simulink model "ejemplo_arduino2"  (R2014b)
settings: Solver=ode3  StartTime=0.0  StopTime=inf  FixedStep=0.001  RelTol=1e-3
libraries: simulink x48, simulink_extras x36, dspswit3 x16, LibrarySimulinkSAS x2, vrlib x2, sldrtlib x1
(part 1 of 2)
settings Model: Creator=Usuario  LastModifiedBy=santd
settings OptimizationCC: UseDivisionForNetSlopeComputation=off  SimCompilerOptimization=off
settings DebuggingCC: FrameProcessingCompatibilityMsg=error
settings RTWCC: RTWCompilerOptimization=off
settings ConfigComp: CovMetricSettings=dw  CovHtmlReporting=on  CovSaveCumulativeToWorkspaceVar=on  CovSaveSingleToWorkspaceVar=on  CovModelRefEnable=Off  CovExternalEMLEnable=off  CovSFcnEnable=off
settings ConfigurationSet: Description=Simscape Multibody

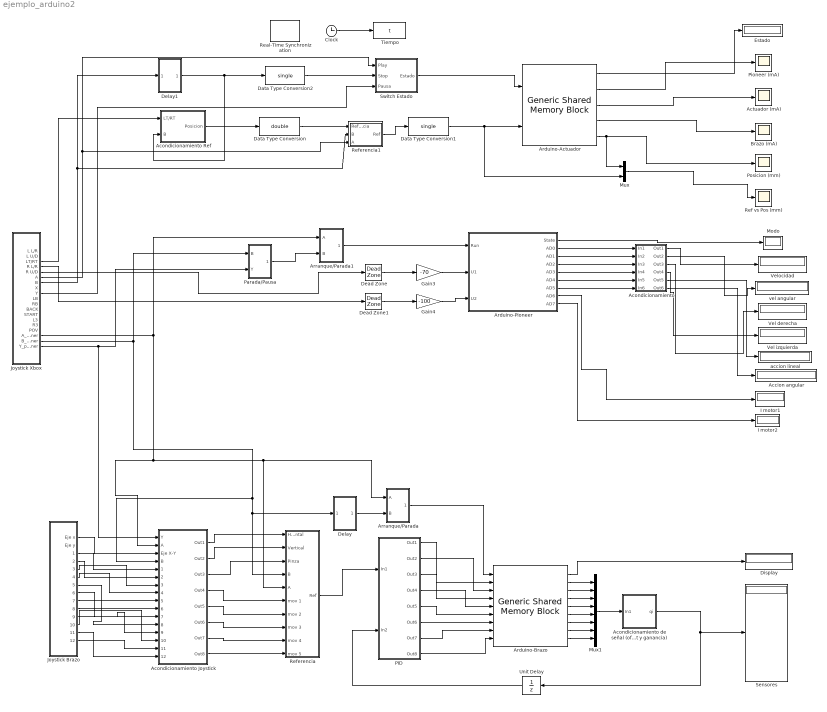
== system ejemplo_arduino2 ==
  Accion angular : Display
  "Acondicionamiento " : Subsystem
  Acondicionamiento Joystick : Subsystem
  Acondicionamiento Ref : Subsystem
  Acondicionamiento de señal (offset y ganancia) : Subsystem
  Actuador (mA) : Scope
      settings: YMin=0  YMax=2000
  Arduino-Actuador : LibrarySimulinkSAS/Generic Shared Memory Block  nombre='memoriaEjemplo'  dispositivo=10  vecE=[3 2 1]  vecS=[4 5 6 156]  tipoE=['f' 'I' 'c']  tipoS=['C' 'i' 'd' 'd']
  Arduino-Brazo : LibrarySimulinkSAS/Generic Shared Memory Block  nombre='memoriaEjemplo'  dispositivo=10  vecE=[3 2 1]  vecS=[4 5 6 156]  tipoE=['f' 'I' 'c']  tipoS=['C' 'i' 'd' 'd']
  Arduino-Pioneer : Subsystem  mask{dev=3}
      mask prompts: dev "Device Number"
      mask Help:
      | HELP DEVICE
      | 
      | - App for using the kit arduino UNO plus Adafruit motor shield 1.2 based on two L293D chips forming 4 H-Bridges. L293D chipset provides 0.6A per bridge (1.2A peak) with thermal shutdown protection, internal kickback protection diodes. Can run motors on 4.5VDC to 25VDC. The shield is compatible with Arduino Mega 1280 & 2560, Diecimila, Duemilanove, and UNO
      | 
      | HELP DRIVERS
      | 
      | Upload the firmware 'Arduino_motor_firmware' in your Arduino UNO kit available from folder '\SAS TOOLS\Software arduino_motor V1.1.0'
      | -------------------------------------------------------------------------------------------------------------------------------------------------------
      | HELP APP
      | 
      | Before running the Simulink model initiate communication with the device through the application 'Arduino_motor.exe' available from folder '\SAS TOOLS\Software arduino_motor V1.1.0'. After executing the program the app icon is available in the taskbar.
      | The app "arduino_motor.exe" is handled from right-click on the icon and selecting the corresponding option:
      | "Play" -> Start the commnunication between the device and the app
      | "Stop" -> Stop the communication
      | "Monitor"->view the state of sensors and communication
      | 
      | -------------------------------------------------------------------------------------------------------------------------------------------------------
      | 
      | HELP BLOCK
      | 
      | Input Ports
      | 
      | Port 'Run': 1 for running and 0 for stopping
      | 
      | Port 'U1': value between [-255;255] which drives the tension applied to the motor 1 of the shield motor Adafruit 1.0
      | Port 'U2': value between [-255;255] which drives the tension applied to the motor 2 of the shield motor Adafruit 1.0
      | Port 'U3': value between [-255;255] which drives the tension applied to the motor 3 of the shield motor Adafruit 1.0
      | Port 'U4': value between [-255;255] which drives the tension applied to the motor 4 of the shield motor Adafruit 1.0
      | 
      | The range [-255;255] is related with the tension range [-V;V], where V is the tension source applied to the motor shield
      | 
      | Output Ports
      | 
      | Port 'State': information about the system. Run=1; Stop=0
      | 
      | Port 'AD0': value between [0;1023] measured in the pin AD0 of the Arduino UNO board
      | Port 'AD1': value between [0;1023] measured in the pin AD1 of the Arduino UNO board
      | Port 'AD2': value between [0;1023] measured in the pin AD2 of the Arduino UNO board
      | Port 'AD3': value between [0;1023] measured in the pin AD3 of the Arduino UNO board
      | 
      | The range [0;1023] is related with the tension range [0;5V] readed on the pins of the Arduino kit A/D conversor
      | -------------------------------------------------------------------------------------------------------------------------------------------------------
      | 
      | HELP SHARE MEMORY (information only for external applications different to "Arduino_motor.exe")
      | 
      | Shared Memory Names:
      | 
      | 'ARDUINO_entrada_'#dev
      | 'ARDUINO_salida_'#dev
      | NOTE: replace #dev with the device number
      mask DialogControl DescGroupVar Prompt: Arduino motor shield
      mask DialogControl DescTextVar Prompt: This block is used to receive and send data via USB port between a UNO Arduino board and the App "Arduino_motor.exe" available on folder '\SAS TOOLS\Software Arduino_motor V1.1.0'. You must upload the firmware "Arduino_motor_firmware" into your Arduino board. More information in Help button.
      mask Display:
      | image('motor_shield.png')
      | color('red')
      | port_label('input',1,'run')
      | port_label('input',2,'U1')
      | port_label('input',3,'U2')
      | port_label('input',4,'U3')
      | port_label('input',5,'U4')
      | color('blue')
      | port_label('output',1,'state')
      | port_label('output',2,'AD0')
      | port_label('output',3,'AD1')
      | port_label('output',4,'AD2')
      | port_label('output',5,'AD3')
  Arranque/Parada : Subsystem
  Arranque/Parada1 : Subsystem
  Brazo (mA) : Scope
      settings: YMin=0  YMax=2000
  Clock : Clock
  Data Type Conversion : DataTypeConversion  OutDataTypeStr=double
  Data Type Conversion1 : DataTypeConversion  OutDataTypeStr=single
  Data Type Conversion2 : DataTypeConversion  OutDataTypeStr=single
  Dead Zone : DeadZone  LowerValue=-0.2  UpperValue=0.2  SaturateOnIntegerOverflow=on
  Dead Zone1 : DeadZone  LowerValue=-0.2  UpperValue=0.2  SaturateOnIntegerOverflow=on
  Delay : Subsystem
  Delay1 : Subsystem
  Display : Display
  Estado : Display
  Gain3 : Gain  Gain=-70  OutDataTypeStr=single
  Gain4 : Gain  Gain=-100  OutDataTypeStr=single
  I motor1 : Display
  I motor2 : Display
  Joystick Brazo : Subsystem
  Joystick Xbox : Subsystem
  Modo : Display
  Mux : Mux  Inputs=2
  Mux1 : Mux  Inputs=8
  PID : Subsystem
  Parada/Pausa : Subsystem
  Pioneer (mA) : Scope
      settings: YMin=0  YMax=2500
  Posicion (mm) : Scope
      settings: YMin=-10  YMax=220
  Real-Time Synchronization : sldrtlib/Real-Time Synchronization
  Ref vs Pos (mm) : Scope
      settings: YMin=0  YMax=200
  Referencia : Subsystem
  Referencia1 : Subsystem
  Sensores : Display
  Switch Estado : Subsystem
  Tiempo : ToWorkspace  VariableName=t  SampleTime=-1
  Unit Delay : UnitDelay  SampleTime=-1
  Vel derecha : Display
  Vel izquierda : Display
  Velocidad : Display
  accion lineal : Display
  vel angular : Display
  wires:
  Clock/1 -> Tiempo/1
  Arduino-Actuador/1 -> Estado/1
  Arduino-Actuador/2 -> Pioneer (mA)/1
  Arduino-Actuador/3 -> Actuador (mA)/1
  Arduino-Actuador/4 -> Brazo (mA)/1
  Joystick Xbox/6(A) -> Referencia1/3(A), Switch Estado/1(Play)
  Joystick Xbox/9(Y) -> Switch Estado/3(Pausa)
  Switch Estado/1(Estado) -> Arduino-Actuador/1
  Arduino-Brazo/1 -> Display/1
  Arduino-Brazo/2 -> Mux1/1
  Arduino-Brazo/9 -> Mux1/8
  Arduino-Brazo/7 -> Mux1/6
  Arduino-Brazo/8 -> Mux1/7
  Arduino-Brazo/6 -> Mux1/5
  Arduino-Brazo/3 -> Mux1/2
  Arduino-Brazo/4 -> Mux1/3
  Arduino-Brazo/5 -> Mux1/4
  Mux1/1 -> Acondicionamiento de señal (offset y ganancia)/1(In1)
  Acondicionamiento de señal (offset y ganancia)/1(qi) -> Unit Delay/1, Sensores/1
  Referencia/1(Ref) -> PID/1(In1)
  Joystick Xbox/17(A_Pionner) -> Arranque/Parada1/1(A), Referencia/5(A), Arranque/Parada/1(A), Acondicionamiento Joystick/2(A)
  Joystick Xbox/18(B_Pionner) -> Parada/Pausa/1(B), Referencia/4(B), Delay/1(In1), Acondicionamiento Joystick/4(B)
  Joystick Xbox/19(Y_pionner) -> Acondicionamiento Joystick/1(Y), Parada/Pausa/2(Y)
  Gain4/1 -> Arduino-Pioneer/3(U2)
  Arduino-Pioneer/1(State) -> Modo/1
  Arranque/Parada1/1(Modo) -> Arduino-Pioneer/1(Run)
  Gain3/1 -> Arduino-Pioneer/2(U1)
  Arduino-Pioneer/8(AD6) -> I motor1/1
  Arduino-Pioneer/9(AD7) -> I motor2/1
  Unit Delay/1 -> PID/2(In2)
  PID/1(Out1) -> Arduino-Brazo/2
  PID/2(Out2) -> Arduino-Brazo/3
  PID/3(Out3) -> Arduino-Brazo/4
  PID/4(Out4) -> Arduino-Brazo/5
  PID/5(Out5) -> Arduino-Brazo/6
  PID/6(Out6) -> Arduino-Brazo/7
  PID/7(Out7) -> Arduino-Brazo/8
  PID/8(Out8) -> Arduino-Brazo/9
  Parada/Pausa/1(Out1) -> Arranque/Parada1/2(B)
  Arduino-Pioneer/2(AD0) -> "Acondicionamiento "/1(In1)
  Arduino-Pioneer/3(AD1) -> "Acondicionamiento "/2(In2)
  Arduino-Pioneer/4(AD2) -> "Acondicionamiento "/3(In3)
  Arduino-Pioneer/5(AD3) -> "Acondicionamiento "/4(In4)
  Arduino-Pioneer/6(AD4) -> "Acondicionamiento "/5(In5)
  Arduino-Pioneer/7(AD5) -> "Acondicionamiento "/6(In6)
  "Acondicionamiento "/1(Out1) -> Velocidad/1
  "Acondicionamiento "/2(Out2) -> vel angular/1
  "Acondicionamiento "/3(Out3) -> Vel derecha/1
  "Acondicionamiento "/4(Out4) -> Vel izquierda/1
  "Acondicionamiento "/5(Out5) -> accion lineal/1
  "Acondicionamiento "/6(Out6) -> Accion angular/1
  Arranque/Parada/1(Modo) -> Arduino-Brazo/1
  Delay/1(Out1) -> Arranque/Parada/2(B)
  Joystick Brazo/1(Eje x) -> Acondicionamiento Joystick/3(Eje X-Y)
  Joystick Brazo/3(1) -> Acondicionamiento Joystick/5(1)
  Joystick Brazo/4(2) -> Acondicionamiento Joystick/6(2)
  Joystick Brazo/5(3) -> Acondicionamiento Joystick/7(3)
  Joystick Brazo/6(4) -> Acondicionamiento Joystick/8(4)
  Joystick Brazo/11(9) -> Acondicionamiento Joystick/13(9)
  Joystick Brazo/12(10) -> Acondicionamiento Joystick/14(10)
  Acondicionamiento Joystick/1(Out1) -> Referencia/1(Horizontal)
  Acondicionamiento Joystick/2(Out2) -> Referencia/2(Vertical)
  Acondicionamiento Joystick/3(Out3) -> Referencia/3(Pinza)
  Acondicionamiento Joystick/4(Out4) -> Referencia/6(mov 1)
  Acondicionamiento Joystick/5(Out5) -> Referencia/7(mov 2)
  Acondicionamiento Joystick/6(Out6) -> Referencia/8(mov 3)
  Acondicionamiento Joystick/7(Out7) -> Referencia/9(mov 4)
  Acondicionamiento Joystick/8(Out8) -> Referencia/10(mov 5)
  Joystick Brazo/9(7) -> Acondicionamiento Joystick/9(5)
  Joystick Brazo/10(8) -> Acondicionamiento Joystick/10(6)
  Joystick Brazo/7(5) -> Acondicionamiento Joystick/12(8)
  Joystick Brazo/8(6) -> Acondicionamiento Joystick/11(7)
  Joystick Brazo/13(11) -> Acondicionamiento Joystick/16(12)
  Joystick Brazo/14(12) -> Acondicionamiento Joystick/15(11)
  Dead Zone1/1 -> Gain4/1
  Dead Zone/1 -> Gain3/1
  Joystick Xbox/4(R L/R) -> Dead Zone1/1
  Joystick Xbox/5(R U/D) -> Dead Zone/1
  Arduino-Actuador/5 -> Posicion (mm)/1, Mux/1
  Joystick Xbox/3(LT/RT) -> Acondicionamiento Ref/1(LT/RT)
  Referencia1/1(Ref) -> Data Type Conversion1/1
  Mux/1 -> Ref vs Pos (mm)/1
  Acondicionamiento Ref/1(Posicion) -> Data Type Conversion/1
  Data Type Conversion/1 -> Referencia1/1(Referencia)
  Data Type Conversion1/1 -> Mux/2, Arduino-Actuador/2
  Joystick Xbox/7(B) -> Delay1/1(In1), Referencia1/2(B)
  Data Type Conversion2/1 -> Switch Estado/2(Stop)
  Delay1/1(Out1) -> Acondicionamiento Ref/2(B), Data Type Conversion2/1

== system ejemplo_arduino2/Acondicionamiento  ==
  In1 : Inport
  In2 : Inport  Port=2
  In3 : Inport  Port=3
  In4 : Inport  Port=4
  In5 : Inport  Port=5
  In6 : Inport  Port=6
  Subsystem : Subsystem
  Subsystem1 : Subsystem
  Subsystem2 : Subsystem
  Subsystem3 : Subsystem
  Subsystem4 : Subsystem
  Subsystem5 : Subsystem
  Out1 : Outport
  Out2 : Outport  Port=2
  Out3 : Outport  Port=3
  Out4 : Outport  Port=4
  Out5 : Outport  Port=5
  Out6 : Outport  Port=6
  wires:
  In4/1 -> Subsystem2/1(In1)
  In3/1 -> Subsystem1/1(In1)
  In2/1 -> Subsystem3/1(In1)
  Subsystem5/1(Out1) -> Out6/1
  In6/1 -> Subsystem5/1(In1)
  Subsystem4/1(Out1) -> Out5/1
  In5/1 -> Subsystem4/1(In1)
  Subsystem2/1(Out1) -> Out4/1
  Subsystem3/1(Out1) -> Out2/1
  Subsystem1/1(Out1) -> Out3/1
  Subsystem/1(Out1) -> Out1/1
  In1/1 -> Subsystem/1(In1)

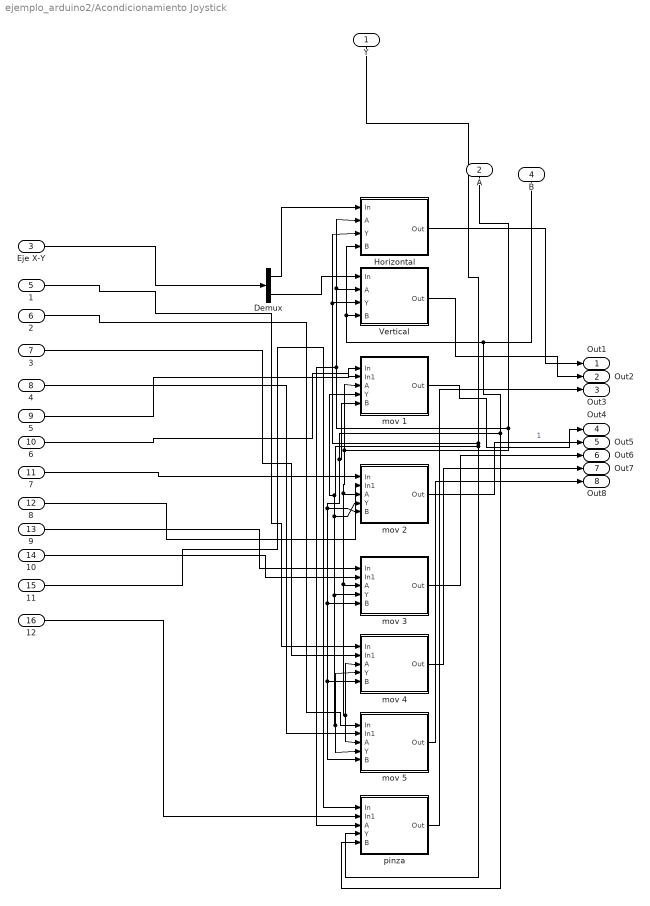
== system ejemplo_arduino2/Acondicionamiento Joystick ==
  Y : Inport
  A : Inport  Port=2
  Eje X-Y : Inport  Port=3
  B : Inport  Port=4
  1 : Inport  Port=5
  2 : Inport  Port=6
  3 : Inport  Port=7
  4 : Inport  Port=8
  5 : Inport  Port=9
  6 : Inport  Port=10
  7 : Inport  Port=11
  8 : Inport  Port=12
  9 : Inport  Port=13
  10 : Inport  Port=14
  11 : Inport  Port=15
  12 : Inport  Port=16
  Demux : Demux  Outputs=2
  Horizontal : Subsystem
  Vertical : Subsystem
  mov 1 : Subsystem
  mov 2 : Subsystem
  mov 3 : Subsystem
  mov 4 : Subsystem
  mov 5 : Subsystem
  pinza : Subsystem
  Out1 : Outport
  Out2 : Outport  Port=2
  Out3 : Outport  Port=3
  Out4 : Outport  Port=4
  Out5 : Outport  Port=5
  Out6 : Outport  Port=6
  Out7 : Outport  Port=7
  Out8 : Outport  Port=8
  wires:
  pinza/1(Out) -> Out3/1
  Eje X-Y/1 -> Demux/1
  11/1 -> pinza/1(In)
  12/1 -> pinza/2(In1)
  mov 1/1(Out) -> Out4/1
  mov 2/1(Out) -> Out5/1  "1"
  mov 3/1(Out) -> Out6/1
  mov 4/1(Out) -> Out7/1
  5/1 -> mov 1/1(In)
  6/1 -> mov 1/2(In1)
  7/1 -> mov 2/1(In)
  8/1 -> mov 2/2(In1)
  9/1 -> mov 3/1(In)
  10/1 -> mov 3/2(In1)
  mov 5/1(Out) -> Out8/1
  Horizontal/1(Out) -> Out1/1
  Vertical/1(Out) -> Out2/1
  Demux/1 -> Horizontal/1(In)
  Demux/2 -> Vertical/1(In)
  1/1 -> mov 4/1(In)
  3/1 -> mov 4/2(In1)
  2/1 -> mov 5/1(In)
  4/1 -> mov 5/2(In1)
  Y/1 -> pinza/4(Y), mov 5/4(Y), mov 4/4(Y), mov 3/4(Y), mov 2/4(Y), mov 1/4(Y), Horizontal/3(Y), Vertical/3(Y)
  A/1 -> Horizontal/2(A), Vertical/2(A), pinza/3(A), mov 5/3(A), mov 4/3(A), mov 3/3(A), mov 2/3(A), mov 1/3(A)
  B/1 -> Horizontal/4(B), Vertical/4(B), mov 5/5(B), mov 4/5(B), mov 3/5(B), mov 2/5(B), mov 1/5(B), pinza/5(B)

== system ejemplo_arduino2/Acondicionamiento Ref ==
  LT/RT : Inport
  B : Inport  Port=2
  Constant : Constant  Value=0
  Data Type Conversion : DataTypeConversion
  Data Type Conversion1 : DataTypeConversion  OutDataTypeStr=single
  Gain : Gain  Gain=-26  OutDataTypeStr=single
  Integrator Limited : Integrator  ExternalReset=level  InitialConditionSource=external  LimitOutput=on  UpperSaturationLimit=200  LowerSaturationLimit=0
  Posicion : Outport
  wires:
  LT/RT/1 -> Gain/1
  Gain/1 -> Data Type Conversion/1
  Data Type Conversion/1 -> Integrator Limited/1
  Integrator Limited/1 -> Data Type Conversion1/1
  Data Type Conversion1/1 -> Posicion/1
  B/1 -> Integrator Limited/2
  Constant/1 -> Integrator Limited/3

== system ejemplo_arduino2/Acondicionamiento de señal (offset y ganancia) ==
  In1 : Inport
  Ganancia : Gain  Gain=diag([0.2022 0.2057 0.2093 0.2047 0.2179 0.2024 0.1931 0.3141])  Multiplication=Matrix(K*u) (u vector)
  Offset : Constant  Value=[-132 -113 -162 -88 -125 -124 -90 -386]
  Sum : Sum  Inputs=|++
  qi : Outport
  wires:
  In1/1 -> Sum/1
  Sum/1 -> Ganancia/1
  Offset/1 -> Sum/2
  Ganancia/1 -> qi/1

== system ejemplo_arduino2/Arduino-Pioneer ==
  Run : Inport
  U1 : Inport  Port=2
  U2 : Inport  Port=3
  Generic Shared Memory Block : S-Function  FunctionName=matlabGenericSHM  Parameters=nombre,dispositivo,vecE,vecS,tipoE,tipoS  EnableBusSupport=off  mask(Generic Share Memory block V2.0){nombre='ARDUINO', dispositivo=3, vecE=[1 1 1], vecS=[1 1 1 1 1 1 1 1 1], tipoE=['f' 'f' 'f'], tipoS=['f' 'f' 'f' 'f' 'f' 'f' 'f' 'f' 'f' ]}
      mask prompts: nombre "Share Memory base name"; dispositivo "Device Number"; vecE "Sizes input vector"; vecS "Sizes output vector"; tipoE "Data Types Inputs"; tipoS "Data Types Outputs"
      mask help:
      | This block allows Simulink communication with external processes through shared memory. It works on Unix and Windows.
      | More information in Help.
      mask Help:
      | Share Memory base name (nombre): It's the base string of share memory ej 'robot'
      | Device Number (dispositivo): integer that identifies the device between multiple in use
      | Two shared memorys are created with names:
      | "%name_entrada_%dispositivo" for the device input (writing)
      | "%name_salida_%dispositivo" for the device output (reading)
      | Sizes input vector (vecE)  : array that specify the number of inputs (array dimension) and the inputs size (array values)
      | Sizes output vector  (vecS): array that specify the number of outputs (array dimension) and the outputs size (array values)
      | Data types input(tipoE): char array that specify each input types
      | Data types output (tipoS): char array that specify each output types
      | Allowed types are:
      | ('f'=float, 'd'=double, 'i'=int32, 'c'=char, 'C'= unsigned char, 'I'=unsigned int)
      | Example.
      | Suppose the following parameters:
      | nombre='exampleMemory'
      | dispositivo=10
      | vecE=[3 2 1]
      | vecS=[6 5 7 8]
      | tipoE=['f' 'I' 'c']
      | tipoS=['C' 'i' 'd' 'd']
      | 
      | Two Share Memories are created with names:
      | "exampleMemory_entrada_10" (block input)
      | "exampleMemory_salida_10"  (block output)
      | 3 inputs are created:
      |  1° Dimension 3, type "unsigned char"
      |  2° Dimension 2, type "int"
      |  3° Dimension 1, type "char"
      | 4 outputs are created:
      |  1° Dimension 6, type "float"
      |  2° Dimension 5, type "unsigned int"
      |  3° Dimension 7, type "double"
      |  3° Dimension 8, type "double"
      mask Display: image('shmem.jpg')
  State : Outport
  AD0 : Outport  Port=2
  AD1 : Outport  Port=3
  AD2 : Outport  Port=4
  AD3 : Outport  Port=5
  AD4 : Outport  Port=6
  AD5 : Outport  Port=7
  AD6 : Outport  Port=8
  AD7 : Outport  Port=9
  wires:
  Generic Shared Memory Block/5 -> AD3/1
  Generic Shared Memory Block/4 -> AD2/1
  Generic Shared Memory Block/3 -> AD1/1
  Generic Shared Memory Block/2 -> AD0/1
  Generic Shared Memory Block/1 -> State/1
  U2/1 -> Generic Shared Memory Block/3
  U1/1 -> Generic Shared Memory Block/2
  Run/1 -> Generic Shared Memory Block/1
  Generic Shared Memory Block/9 -> AD7/1
  Generic Shared Memory Block/8 -> AD6/1
  Generic Shared Memory Block/7 -> AD5/1
  Generic Shared Memory Block/6 -> AD4/1

== system ejemplo_arduino2/Arranque//Parada ==
  A : Inport
  B : Inport  Port=2
  Data Type Conversion2 : DataTypeConversion  OutDataTypeStr=single
  Detect Rise Positive : simulink/Logic and Bit Operations/Detect Rise Positive  vinit=0  InputProcessing=Inherited  OutDataTypeStr=boolean
  Detect Rise Positive1 : simulink/Logic and Bit Operations/Detect Rise Positive  vinit=0  InputProcessing=Inherited  OutDataTypeStr=boolean
  Entrada : Display
  S-R Flip-Flop : simulink_extras/Flip Flops/S-R Flip-Flop  initial_condition=0
  Modo : Outport
  wires:
  B/1 -> Detect Rise Positive1/1
  S-R Flip-Flop/1 -> Entrada/1, Data Type Conversion2/1
  Detect Rise Positive/1 -> S-R Flip-Flop/1
  Data Type Conversion2/1 -> Modo/1
  Detect Rise Positive1/1 -> S-R Flip-Flop/2
  A/1 -> Detect Rise Positive/1

== system ejemplo_arduino2/Arranque//Parada1 ==
  A : Inport
  B : Inport  Port=2
  Data Type Conversion2 : DataTypeConversion  OutDataTypeStr=single
  Detect Rise Positive : simulink/Logic and Bit Operations/Detect Rise Positive  vinit=0  InputProcessing=Inherited  OutDataTypeStr=boolean
  Detect Rise Positive1 : simulink/Logic and Bit Operations/Detect Rise Positive  vinit=0  InputProcessing=Inherited  OutDataTypeStr=boolean
  Entrada : Display
  S-R Flip-Flop : simulink_extras/Flip Flops/S-R Flip-Flop  initial_condition=0
  Modo : Outport
  wires:
  B/1 -> Detect Rise Positive1/1
  S-R Flip-Flop/1 -> Entrada/1, Data Type Conversion2/1
  Detect Rise Positive/1 -> S-R Flip-Flop/1
  Data Type Conversion2/1 -> Modo/1
  Detect Rise Positive1/1 -> S-R Flip-Flop/2
  A/1 -> Detect Rise Positive/1

== system ejemplo_arduino2/Delay ==
  In1 : Inport
  Data Type Conversion : DataTypeConversion
  Data Type Conversion1 : DataTypeConversion
  Transport Delay : TransportDelay  DelayTime=2  InitialOutput=1
  Out1 : Outport
  wires:
  In1/1 -> Data Type Conversion/1
  Data Type Conversion/1 -> Transport Delay/1
  Transport Delay/1 -> Data Type Conversion1/1
  Data Type Conversion1/1 -> Out1/1

== system ejemplo_arduino2/Delay1 ==
  In1 : Inport
  Data Type Conversion : DataTypeConversion
  Data Type Conversion1 : DataTypeConversion
  Transport Delay : TransportDelay  DelayTime=4  InitialOutput=1
  Out1 : Outport
  wires:
  In1/1 -> Data Type Conversion/1
  Data Type Conversion/1 -> Transport Delay/1
  Transport Delay/1 -> Data Type Conversion1/1
  Data Type Conversion1/1 -> Out1/1

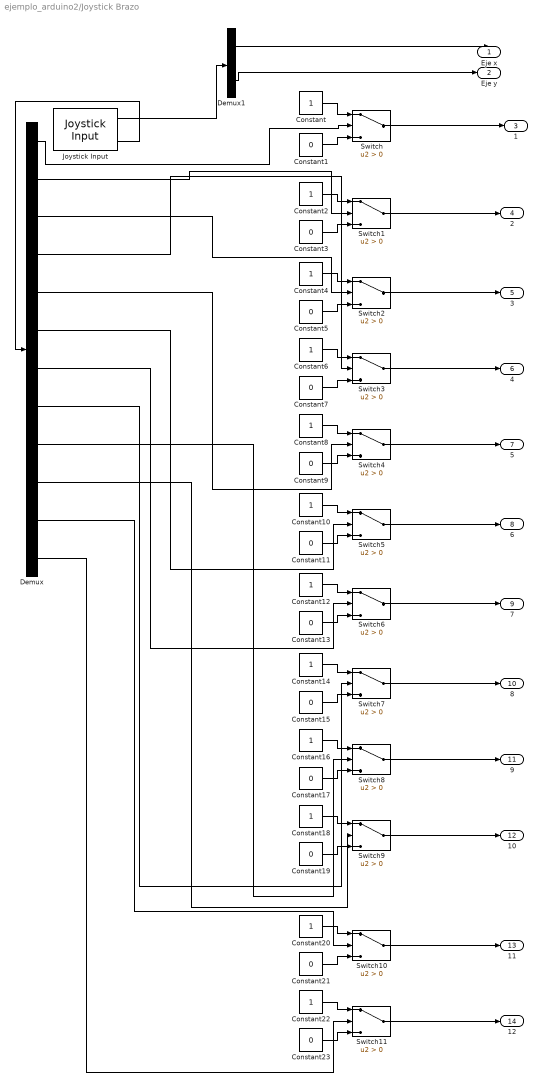
== system ejemplo_arduino2/Joystick Brazo ==
  Constant{,2,4,6,8,10,12,14,16,18,20,22} (12 alike) : Constant
  Constant{1,3,5,7,9,11,13,15,17,19,21,23} (12 alike) : Constant  Value=0
  Demux : Demux  Outputs=12
  Demux1 : Demux  Outputs=2
  Joystick Input : vrlib/Joystick Input  joyid=1  adjustports=off  forcefeed=off
  Switch{,1..11} (12 alike) : Switch  Criteria=u2 > Threshold  OutDataTypeStr=single  InputSameDT=on
  Eje x : Outport
  Eje y : Outport  Port=2
  1 : Outport  Port=3
  2 : Outport  Port=4
  3 : Outport  Port=5
  4 : Outport  Port=6
  5 : Outport  Port=7
  6 : Outport  Port=8
  7 : Outport  Port=9
  8 : Outport  Port=10
  9 : Outport  Port=11
  10 : Outport  Port=12
  11 : Outport  Port=13
  12 : Outport  Port=14
  wires:
  Joystick Input/2 -> Demux/1
  Demux/4 -> Switch3/2
  Demux/5 -> Switch4/2
  Constant16/1 -> Switch8/1
  Constant18/1 -> Switch9/1
  Demux/2 -> Switch1/2
  Switch9/1 -> 10/1
  Constant19/1 -> Switch9/3
  Switch8/1 -> 9/1
  Constant17/1 -> Switch8/3
  Demux/1 -> Switch/2
  Constant6/1 -> Switch3/1
  Constant3/1 -> Switch1/3
  Demux1/1 -> Eje x/1
  Demux/10 -> Switch9/2
  Demux/9 -> Switch8/2
  Switch2/1 -> 3/1
  Constant14/1 -> Switch7/1
  Switch7/1 -> 8/1
  Constant2/1 -> Switch1/1
  Constant5/1 -> Switch2/3
  Demux/8 -> Switch7/2
  Demux/7 -> Switch6/2
  Switch1/1 -> 2/1
  Constant4/1 -> Switch2/1
  Constant15/1 -> Switch7/3
  Constant7/1 -> Switch3/3
  Switch3/1 -> 4/1
  Demux/3 -> Switch2/2
  Constant10/1 -> Switch5/1
  Switch6/1 -> 7/1
  Switch5/1 -> 6/1
  Constant12/1 -> Switch6/1
  Constant13/1 -> Switch6/3
  Demux/6 -> Switch5/2
  Constant11/1 -> Switch5/3
  Switch/1 -> 1/1
  Constant8/1 -> Switch4/1
  Demux1/2 -> Eje y/1
  Constant9/1 -> Switch4/3
  Switch4/1 -> 5/1
  Constant1/1 -> Switch/3
  Constant/1 -> Switch/1
  Joystick Input/1 -> Demux1/1
  Constant20/1 -> Switch10/1
  Constant22/1 -> Switch11/1
  Switch11/1 -> 12/1
  Constant23/1 -> Switch11/3
  Switch10/1 -> 11/1
  Constant21/1 -> Switch10/3
  Demux/11 -> Switch10/2
  Demux/12 -> Switch11/2

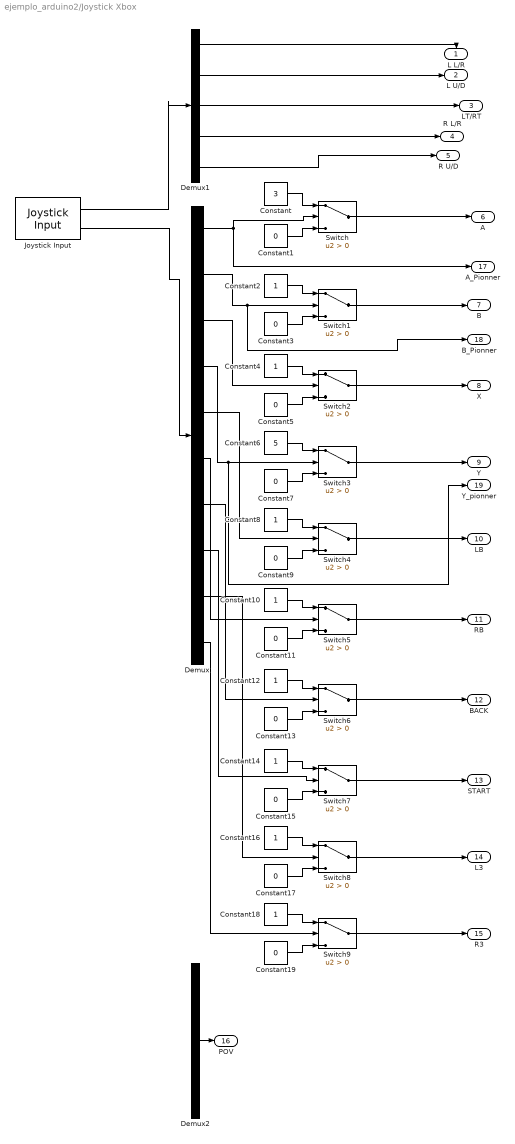
== system ejemplo_arduino2/Joystick Xbox ==
  Constant : Constant  Value=3
  Constant{1,3,5,7,9,11,13,15,17,19} (10 alike) : Constant  Value=0
  Constant{2,4,8,10,12,14,16,18} (8 alike) : Constant
  Constant6 : Constant  Value=5
  Demux : Demux  Outputs=10
  Demux1 : Demux  Outputs=5
  Demux2 : Demux  Outputs=1
  Joystick Input : vrlib/Joystick Input  joyid=1  adjustports=off  forcefeed=off
  Switch{,1..9} (10 alike) : Switch  Criteria=u2 > Threshold  OutDataTypeStr=single  InputSameDT=on
  L L/R : Outport
  L U/D : Outport  Port=2
  LT/RT : Outport  Port=3
  R L/R : Outport  Port=4
  R U/D : Outport  Port=5
  A : Outport  Port=6
  B : Outport  Port=7
  X : Outport  Port=8
  Y : Outport  Port=9
  LB : Outport  Port=10
  RB : Outport  Port=11
  BACK : Outport  Port=12
  START : Outport  Port=13
  L3 : Outport  Port=14
  R3 : Outport  Port=15
  POV : Outport  Port=16
  A_Pionner : Outport  Port=17
  B_Pionner : Outport  Port=18
  Y_pionner : Outport  Port=19
  wires:
  Joystick Input/2 -> Demux/1
  Demux2/1 -> POV/1
  ? -> Demux2/1
  Demux/4 -> Y_pionner/1, Switch3/2
  Demux/5 -> Switch4/2
  Constant16/1 -> Switch8/1
  Demux1/4 -> R L/R/1
  Constant18/1 -> Switch9/1
  Demux/2 -> B_Pionner/1, Switch1/2
  Switch9/1 -> R3/1
  Constant19/1 -> Switch9/3
  Switch8/1 -> L3/1
  Constant17/1 -> Switch8/3
  Demux/1 -> A_Pionner/1, Switch/2
  Demux1/5 -> R U/D/1
  Constant6/1 -> Switch3/1
  Constant3/1 -> Switch1/3
  Demux1/1 -> L L/R/1
  Demux/10 -> Switch9/2
  Demux/9 -> Switch8/2
  Switch2/1 -> X/1
  Constant14/1 -> Switch7/1
  Switch7/1 -> START/1
  Constant2/1 -> Switch1/1
  Constant5/1 -> Switch2/3
  Demux/8 -> Switch7/2
  Demux/7 -> Switch6/2
  Switch1/1 -> B/1
  Constant4/1 -> Switch2/1
  Constant15/1 -> Switch7/3
  Constant7/1 -> Switch3/3
  Switch3/1 -> Y/1
  Demux/3 -> Switch2/2
  Constant10/1 -> Switch5/1
  Switch6/1 -> BACK/1
  Switch5/1 -> RB/1
  Constant12/1 -> Switch6/1
  Constant13/1 -> Switch6/3
  Demux/6 -> Switch5/2
  Constant11/1 -> Switch5/3
  Switch/1 -> A/1
  Constant8/1 -> Switch4/1
  Demux1/2 -> L U/D/1
  Constant9/1 -> Switch4/3
  Switch4/1 -> LB/1
  Constant1/1 -> Switch/3
  Constant/1 -> Switch/1
  Joystick Input/1 -> Demux1/1
  Demux1/3 -> LT/RT/1

== system ejemplo_arduino2/PID ==
  In1 : Inport
  In2 : Inport  Port=2
  Demux : Demux  Outputs=8
  PID Controller{1..8} (8 alike) : simulink/Continuous/PID Controller  Controller=PID  TimeDomain=Continuous-time  SampleTime=-1  IntegratorMethod=Forward Euler  FilterMethod=Forward Euler  Form=Parallel  P=1  I=1  D=0  N=100  InitialConditionSource=internal  InitialConditionForIntegrator=0  InitialConditionForFilter=0  ExternalReset=none  LimitOutput=off  UpperSaturationLimit=inf  LowerSaturationLimit=-inf  LinearizeAsGain=on  AntiWindupMode=none  Kb=1  TrackingMode=off  Kt=1  PParamMin=[]  PParamMax=[]  IParamMin=[]  IParamMax=[]  DParamMin=[]  DParamMax=[]  NParamMin=[]  NParamMax=[]  KbParamMin=[]  KbParamMax=[]  KtParamMin=[]  KtParamMax=[]  POutMin=[]  POutMax=[]  IOutMin=[]  IOutMax=[]  DOutMin=[]  DOutMax=[]  NOutMin=[]  NOutMax=[]  KbOutMin=[]  KbOutMax=[]  KtOutMin=[]  KtOutMax=[]  IntegratorOutMin=[]  IntegratorOutMax=[]  FilterOutMin=[]  FilterOutMax=[]  SumOutMin=[]  SumOutMax=[]  SumI1OutMin=[]  SumI1OutMax=[]  SumI2OutMin=[]  SumI2OutMax=[]  SumI3OutMin=[]  SumI3OutMax=[]  SumDOutMin=[]  SumDOutMax=[]  SaturationOutMin=[]  SaturationOutMax=[]  IntegratorContinuousStateAttributes=''  IntegratorStateMustResolveToSignalObject=off  IntegratorRTWStateStorageClass=Auto  FilterContinuousStateAttributes=''  FilterStateMustResolveToSignalObject=off  FilterRTWStateStorageClass=Auto  DifferentiatorICPrevScaledInput=0  DifferentiatorOutMin=[]  DifferentiatorOutMax=[]  UseFilter=on
  Subtract1 : Sum  Inputs=+-
  Out1 : Outport
  Out2 : Outport  Port=2
  Out3 : Outport  Port=3
  Out4 : Outport  Port=4
  Out5 : Outport  Port=5
  Out6 : Outport  Port=6
  Out7 : Outport  Port=7
  Out8 : Outport  Port=8
  wires:
  Subtract1/1 -> Demux/1
  PID Controller2/1 -> Out2/1
  PID Controller3/1 -> Out3/1
  Demux/3 -> PID Controller3/1
  PID Controller1/1 -> Out1/1
  Demux/1 -> PID Controller1/1
  Demux/2 -> PID Controller2/1
  In2/1 -> Subtract1/2
  Demux/7 -> PID Controller7/1
  PID Controller5/1 -> Out5/1
  PID Controller8/1 -> Out8/1
  Demux/5 -> PID Controller5/1
  Demux/6 -> PID Controller6/1
  PID Controller6/1 -> Out6/1
  PID Controller4/1 -> Out4/1
  Demux/4 -> PID Controller4/1
  Demux/8 -> PID Controller8/1
  PID Controller7/1 -> Out7/1
  In1/1 -> Subtract1/1

== system ejemplo_arduino2/Parada//Pausa ==
  B : Inport
  Y : Inport  Port=2
  Add : Sum
  Saturation : Saturate  UpperLimit=1  LowerLimit=0
  Out1 : Outport
  wires:
  Y/1 -> Add/2
  Saturation/1 -> Out1/1
  Add/1 -> Saturation/1
  B/1 -> Add/1

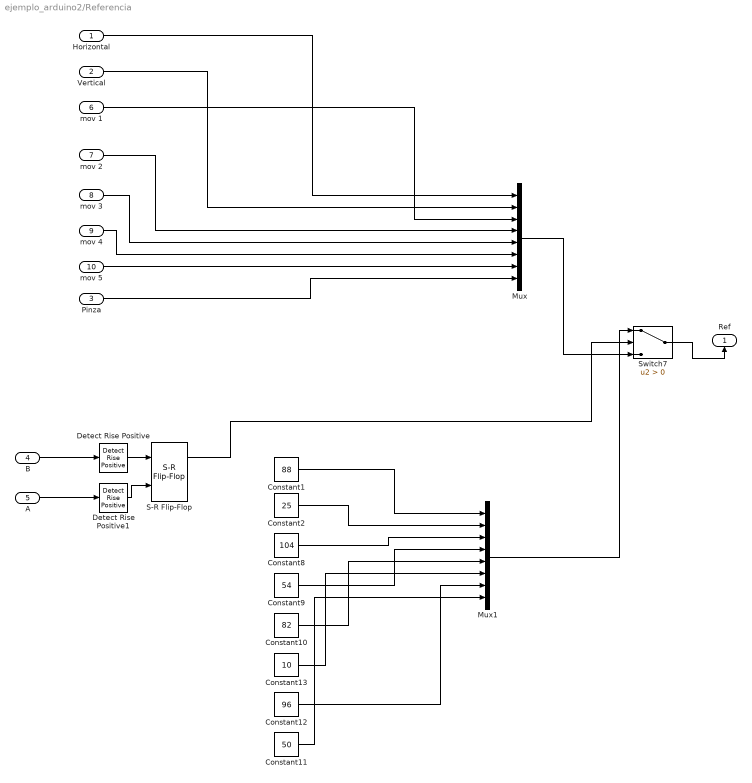
== system ejemplo_arduino2/Referencia ==
  Horizontal : Inport
  Vertical : Inport  Port=2
  Pinza : Inport  Port=3
  B : Inport  Port=4
  A : Inport  Port=5
  mov 1 : Inport  Port=6
  mov 2 : Inport  Port=7
  mov 3 : Inport  Port=8
  mov 4 : Inport  Port=9
  mov 5 : Inport  Port=10
  Constant1 : Constant  Value=88
  Constant10 : Constant  Value=82
  Constant11 : Constant  Value=50
  Constant12 : Constant  Value=96
  Constant13 : Constant  Value=10
  Constant2 : Constant  Value=25
  Constant8 : Constant  Value=104
  Constant9 : Constant  Value=54
  Detect Rise Positive : simulink/Logic and Bit Operations/Detect Rise Positive  vinit=0  InputProcessing=Inherited  OutDataTypeStr=boolean
  Detect Rise Positive1 : simulink/Logic and Bit Operations/Detect Rise Positive  vinit=0  InputProcessing=Inherited  OutDataTypeStr=boolean
  Mux : Mux  Inputs=8
  Mux1 : Mux  Inputs=8
  S-R Flip-Flop : simulink_extras/Flip Flops/S-R Flip-Flop  initial_condition=0
  Switch7 : Switch  Criteria=u2 > Threshold
  Ref : Outport
  wires:
  Pinza/1 -> Mux/8
  Vertical/1 -> Mux/2
  Horizontal/1 -> Mux/1
  Switch7/1 -> Ref/1
  Constant1/1 -> Mux1/1
  Constant2/1 -> Mux1/2
  Constant8/1 -> Mux1/3
  Constant9/1 -> Mux1/4
  Constant10/1 -> Mux1/5
  Constant13/1 -> Mux1/6
  Constant12/1 -> Mux1/7
  Constant11/1 -> Mux1/8
  Mux/1 -> Switch7/3
  Mux1/1 -> Switch7/1
  Detect Rise Positive/1 -> S-R Flip-Flop/1
  Detect Rise Positive1/1 -> S-R Flip-Flop/2
  S-R Flip-Flop/1 -> Switch7/2
  A/1 -> Detect Rise Positive1/1
  B/1 -> Detect Rise Positive/1
  mov 1/1 -> Mux/3
  mov 2/1 -> Mux/4
  mov 3/1 -> Mux/5
  mov 4/1 -> Mux/6
  mov 5/1 -> Mux/7

== system ejemplo_arduino2/Referencia1 ==
  Referencia : Inport
  B : Inport  Port=2
  A : Inport  Port=3
  Constant1 : Constant  Value=0
  Detect Rise Positive : simulink/Logic and Bit Operations/Detect Rise Positive  vinit=0  InputProcessing=Inherited  OutDataTypeStr=boolean
  Detect Rise Positive1 : simulink/Logic and Bit Operations/Detect Rise Positive  vinit=0  InputProcessing=Inherited  OutDataTypeStr=boolean
  S-R Flip-Flop : simulink_extras/Flip Flops/S-R Flip-Flop  initial_condition=0
  Switch7 : Switch  Criteria=u2 > Threshold
  Ref : Outport
  wires:
  Switch7/1 -> Ref/1
  Referencia/1 -> Switch7/3
  Detect Rise Positive/1 -> S-R Flip-Flop/1
  Detect Rise Positive1/1 -> S-R Flip-Flop/2
  S-R Flip-Flop/1 -> Switch7/2
  A/1 -> Detect Rise Positive1/1
  B/1 -> Detect Rise Positive/1
  Constant1/1 -> Switch7/1

== system ejemplo_arduino2/Switch Estado ==
  Play : Inport
  Stop : Inport  Port=2
  Pausa : Inport  Port=3
  Sum : Sum  Inputs=|+++
  Estado : Outport
  wires:
  Play/1 -> Sum/1
  Stop/1 -> Sum/2
  Pausa/1 -> Sum/3
  Sum/1 -> Estado/1

== system ejemplo_arduino2/Acondicionamiento /Subsystem ==
  In1 : Inport
  Gain : Gain  Gain=1/(2*117.02857)
  To Workspace : ToWorkspace  VariableName=vel  SaveFormat=Timeseries  SampleTime=-1
  velocidad lineal : Scope
  Out1 : Outport
  wires:
  Gain/1 -> Out1/1, To Workspace/1, velocidad lineal/1
  In1/1 -> Gain/1

== system ejemplo_arduino2/Acondicionamiento /Subsystem1 ==
  In1 : Inport
  Gain6 : Gain  Gain=1/(2*117.02857)
  To Workspace6 : ToWorkspace  VariableName=vd  SaveFormat=Timeseries  SampleTime=-1
  velocidad lineal1 : Scope
  Out1 : Outport
  wires:
  In1/1 -> Gain6/1
  Gain6/1 -> Out1/1, velocidad lineal1/1, To Workspace6/1

== system ejemplo_arduino2/Acondicionamiento /Subsystem2 ==
  In1 : Inport
  Gain7 : Gain  Gain=1/(2*117.02857)
  To Workspace7 : ToWorkspace  VariableName=vi  SaveFormat=Timeseries  SampleTime=-1
  velocidad lineal2 : Scope
  Out1 : Outport
  wires:
  In1/1 -> Gain7/1
  Gain7/1 -> Out1/1, To Workspace7/1, velocidad lineal2/1

== system ejemplo_arduino2/Acondicionamiento /Subsystem3 ==
  In1 : Inport
  Gain1 : Gain  Gain=1/(2*81.92)  ParamDataTypeStr=double
  To Workspace3 : ToWorkspace  VariableName=wel  SaveFormat=Timeseries  SampleTime=-1
  Out1 : Outport
  wires:
  Gain1/1 -> Out1/1, To Workspace3/1
  In1/1 -> Gain1/1

== system ejemplo_arduino2/Acondicionamiento /Subsystem4 ==
  In1 : Inport
  Gain5 : Gain  Gain=1/(2*682.66)
  To Workspace4 : ToWorkspace  VariableName=uv  SaveFormat=Timeseries  SampleTime=-1
  Out1 : Outport
  wires:
  Gain5/1 -> Out1/1, To Workspace4/1
  In1/1 -> Gain5/1

== system ejemplo_arduino2/Acondicionamiento /Subsystem5 ==
  In1 : Inport
  Gain2 : Gain  Gain=1/(2*682.66)
  To Workspace5 : ToWorkspace  VariableName=uw  SaveFormat=Timeseries  SampleTime=-1
  Out1 : Outport
  wires:
  Gain2/1 -> Out1/1, To Workspace5/1
  In1/1 -> Gain2/1

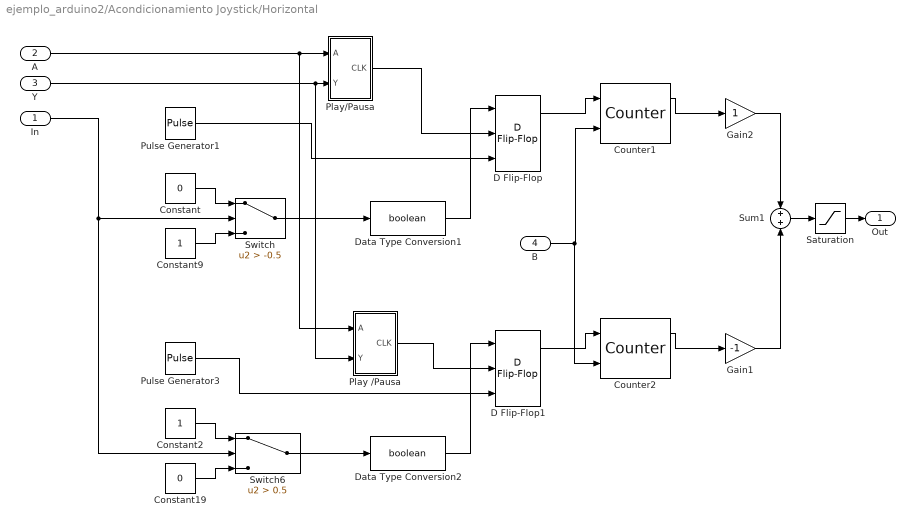
== system ejemplo_arduino2/Acondicionamiento Joystick/Horizontal ==
  In : Inport
  A : Inport  Port=2
  Y : Inport  Port=3
  B : Inport  Port=4
  Constant : Constant  Value=0
  Constant19 : Constant  Value=0
  Constant2 : Constant
  Constant9 : Constant
  Counter1 : dspswit3/Counter  Direction=Up  CountEvent=Rising edge  CounterSize=User defined  MaxCount=255  InitialCount=0  Output=Count and Hit  HitValue=32  ResetInput=on  SamplesPerFrame=1  Ts=1  CntDtype=double  HitDtype=Logical
  Counter2 : dspswit3/Counter  Direction=Up  CountEvent=Rising edge  CounterSize=User defined  MaxCount=255  InitialCount=0  Output=Count and Hit  HitValue=32  ResetInput=on  SamplesPerFrame=1  Ts=1  CntDtype=double  HitDtype=Logical
  D Flip-Flop : simulink_extras/Flip Flops/D Flip-Flop
  D Flip-Flop1 : simulink_extras/Flip Flops/D Flip-Flop
  Data Type Conversion1 : DataTypeConversion  OutDataTypeStr=boolean
  Data Type Conversion2 : DataTypeConversion  OutDataTypeStr=boolean
  Gain1 : Gain  Gain=-1
  Gain2 : Gain
  Play /Pausa : Subsystem
  Play/Pausa : Subsystem
  Pulse Generator1 : DiscretePulseGenerator  PulseType=Time based  Period=0.05  PulseWidth=50
  Pulse Generator3 : DiscretePulseGenerator  PulseType=Time based  Period=0.05  PulseWidth=50
  Saturation : Saturate  UpperLimit=180  LowerLimit=0
  Sum1 : Sum  Inputs=+|+
  Switch : Switch  Criteria=u2 > Threshold  Threshold=-0.5  OutDataTypeStr=single  InputSameDT=on
  Switch6 : Switch  Criteria=u2 > Threshold  Threshold=0.5  OutDataTypeStr=single  InputSameDT=on
  Out : Outport
  wires:
  Counter1/1 -> Gain2/1
  Constant/1 -> Switch/1
  Constant9/1 -> Switch/3
  Constant2/1 -> Switch6/1
  Counter2/1 -> Gain1/1
  Gain1/1 -> Sum1/2
  D Flip-Flop1/1 -> Counter2/1
  Switch6/1 -> Data Type Conversion2/1
  Data Type Conversion2/1 -> D Flip-Flop1/1
  Pulse Generator3/1 -> D Flip-Flop1/3
  Constant19/1 -> Switch6/3
  In/1 -> Switch6/2, Switch/2
  Saturation/1 -> Out/1
  Pulse Generator1/1 -> D Flip-Flop/3
  Sum1/1 -> Saturation/1
  Gain2/1 -> Sum1/1
  D Flip-Flop/1 -> Counter1/1
  Data Type Conversion1/1 -> D Flip-Flop/1
  Switch/1 -> Data Type Conversion1/1
  A/1 -> Play/Pausa/1(A), Play /Pausa/1(A)
  Y/1 -> Play /Pausa/2(Y), Play/Pausa/2(Y)
  Play/Pausa/1(CLK) -> D Flip-Flop/2
  Play /Pausa/1(CLK) -> D Flip-Flop1/2
  B/1 -> Counter2/2, Counter1/2

== system ejemplo_arduino2/Acondicionamiento Joystick/Vertical ==
  In : Inport
  A : Inport  Port=2
  Y : Inport  Port=3
  B : Inport  Port=4
  Constant : Constant  Value=0
  Constant19 : Constant  Value=0
  Constant2 : Constant
  Constant9 : Constant
  Counter1 : dspswit3/Counter  Direction=Up  CountEvent=Rising edge  CounterSize=User defined  MaxCount=255  InitialCount=0  Output=Count and Hit  HitValue=32  ResetInput=on  SamplesPerFrame=1  Ts=1  CntDtype=double  HitDtype=Logical
  Counter2 : dspswit3/Counter  Direction=Up  CountEvent=Rising edge  CounterSize=User defined  MaxCount=255  InitialCount=0  Output=Count and Hit  HitValue=32  ResetInput=on  SamplesPerFrame=1  Ts=1  CntDtype=double  HitDtype=Logical
  D Flip-Flop : simulink_extras/Flip Flops/D Flip-Flop
  D Flip-Flop1 : simulink_extras/Flip Flops/D Flip-Flop
  Data Type Conversion1 : DataTypeConversion  OutDataTypeStr=boolean
  Data Type Conversion2 : DataTypeConversion  OutDataTypeStr=boolean
  Gain1 : Gain  Gain=-1
  Gain2 : Gain
  Play /Pausa : Subsystem
  Play/Pausa : Subsystem
  Pulse Generator1 : DiscretePulseGenerator  PulseType=Time based  Period=0.1  PulseWidth=50
  Pulse Generator3 : DiscretePulseGenerator  PulseType=Time based  Period=0.1  PulseWidth=50
  Saturation : Saturate  UpperLimit=180  LowerLimit=0
  Sum1 : Sum  Inputs=+|+
  Switch : Switch  Criteria=u2 > Threshold  Threshold=-0.5  OutDataTypeStr=single  InputSameDT=on
  Switch6 : Switch  Criteria=u2 > Threshold  Threshold=0.5  OutDataTypeStr=single  InputSameDT=on
  Out : Outport
  wires:
  Counter1/1 -> Gain2/1
  Constant/1 -> Switch/1
  Constant9/1 -> Switch/3
  Constant2/1 -> Switch6/1
  Counter2/1 -> Gain1/1
  Gain1/1 -> Sum1/2
  D Flip-Flop1/1 -> Counter2/1
  Switch6/1 -> Data Type Conversion2/1
  Data Type Conversion2/1 -> D Flip-Flop1/1
  Pulse Generator3/1 -> D Flip-Flop1/3
  Constant19/1 -> Switch6/3
  In/1 -> Switch6/2, Switch/2
  Saturation/1 -> Out/1
  Pulse Generator1/1 -> D Flip-Flop/3
  Sum1/1 -> Saturation/1
  Gain2/1 -> Sum1/1
  D Flip-Flop/1 -> Counter1/1
  Data Type Conversion1/1 -> D Flip-Flop/1
  Switch/1 -> Data Type Conversion1/1
  Play/Pausa/1(CLK) -> D Flip-Flop/2
  Play /Pausa/1(CLK) -> D Flip-Flop1/2
  A/1 -> Play /Pausa/1(A), Play/Pausa/1(A)
  Y/1 -> Play /Pausa/2(Y), Play/Pausa/2(Y)
  B/1 -> Counter1/2, Counter2/2

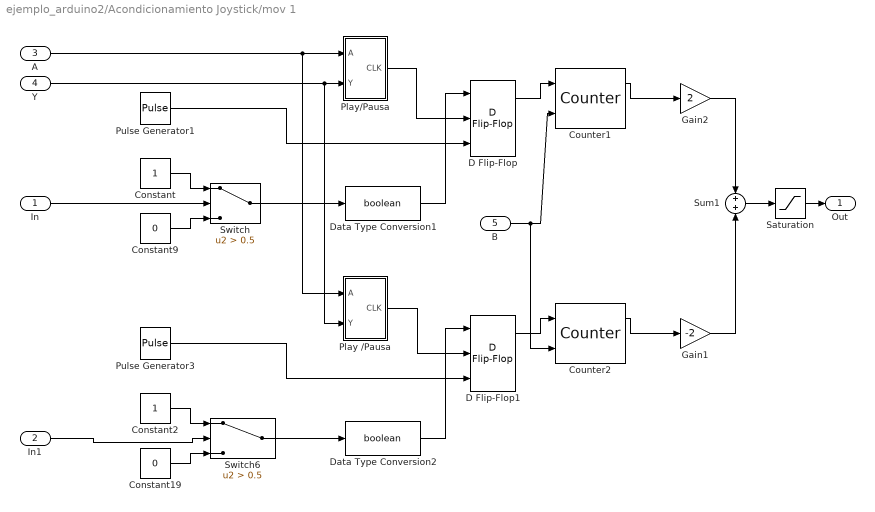
== system ejemplo_arduino2/Acondicionamiento Joystick/mov 1 ==
  In : Inport
  In1 : Inport  Port=2
  A : Inport  Port=3
  Y : Inport  Port=4
  B : Inport  Port=5
  Constant : Constant
  Constant19 : Constant  Value=0
  Constant2 : Constant
  Constant9 : Constant  Value=0
  Counter1 : dspswit3/Counter  Direction=Up  CountEvent=Rising edge  CounterSize=User defined  MaxCount=255  InitialCount=0  Output=Count and Hit  HitValue=32  ResetInput=on  SamplesPerFrame=1  Ts=1  CntDtype=double  HitDtype=Logical
  Counter2 : dspswit3/Counter  Direction=Up  CountEvent=Rising edge  CounterSize=User defined  MaxCount=255  InitialCount=0  Output=Count and Hit  HitValue=32  ResetInput=on  SamplesPerFrame=1  Ts=1  CntDtype=double  HitDtype=Logical
  D Flip-Flop : simulink_extras/Flip Flops/D Flip-Flop
  D Flip-Flop1 : simulink_extras/Flip Flops/D Flip-Flop
  Data Type Conversion1 : DataTypeConversion  OutDataTypeStr=boolean
  Data Type Conversion2 : DataTypeConversion  OutDataTypeStr=boolean
  Gain1 : Gain  Gain=-2
  Gain2 : Gain  Gain=2
  Play /Pausa : Subsystem
  Play/Pausa : Subsystem
  Pulse Generator1 : DiscretePulseGenerator  PulseType=Time based  Period=0.1  PulseWidth=50
  Pulse Generator3 : DiscretePulseGenerator  PulseType=Time based  Period=0.1  PulseWidth=50
  Saturation : Saturate  UpperLimit=180  LowerLimit=0
  Sum1 : Sum  Inputs=+|+
  Switch : Switch  Criteria=u2 > Threshold  Threshold=0.5  OutDataTypeStr=single  InputSameDT=on
  Switch6 : Switch  Criteria=u2 > Threshold  Threshold=0.5  OutDataTypeStr=single  InputSameDT=on
  Out : Outport
  wires:
  Counter1/1 -> Gain2/1
  Constant/1 -> Switch/1
  Constant9/1 -> Switch/3
  Constant2/1 -> Switch6/1
  Counter2/1 -> Gain1/1
  Gain1/1 -> Sum1/2
  D Flip-Flop1/1 -> Counter2/1
  Switch6/1 -> Data Type Conversion2/1
  Data Type Conversion2/1 -> D Flip-Flop1/1
  Pulse Generator3/1 -> D Flip-Flop1/3
  Constant19/1 -> Switch6/3
  In/1 -> Switch/2
  Saturation/1 -> Out/1
  Pulse Generator1/1 -> D Flip-Flop/3
  Sum1/1 -> Saturation/1
  Gain2/1 -> Sum1/1
  D Flip-Flop/1 -> Counter1/1
  Data Type Conversion1/1 -> D Flip-Flop/1
  Switch/1 -> Data Type Conversion1/1
  In1/1 -> Switch6/2
  Play/Pausa/1(CLK) -> D Flip-Flop/2
  Play /Pausa/1(CLK) -> D Flip-Flop1/2
  A/1 -> Play /Pausa/1(A), Play/Pausa/1(A)
  Y/1 -> Play /Pausa/2(Y), Play/Pausa/2(Y)
  B/1 -> Counter1/2, Counter2/2

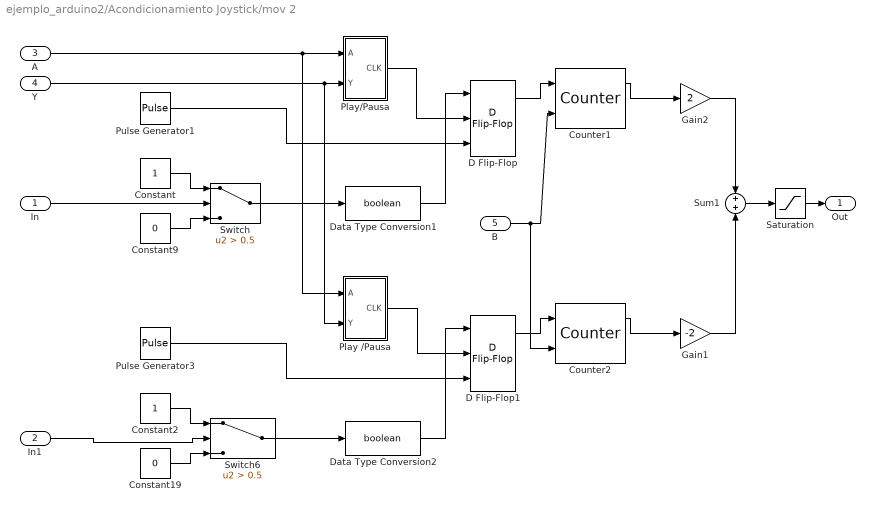
== system ejemplo_arduino2/Acondicionamiento Joystick/mov 2 ==
  In : Inport
  In1 : Inport  Port=2
  A : Inport  Port=3
  Y : Inport  Port=4
  B : Inport  Port=5
  Constant : Constant
  Constant19 : Constant  Value=0
  Constant2 : Constant
  Constant9 : Constant  Value=0
  Counter1 : dspswit3/Counter  Direction=Up  CountEvent=Rising edge  CounterSize=User defined  MaxCount=255  InitialCount=0  Output=Count and Hit  HitValue=32  ResetInput=on  SamplesPerFrame=1  Ts=1  CntDtype=double  HitDtype=Logical
  Counter2 : dspswit3/Counter  Direction=Up  CountEvent=Rising edge  CounterSize=User defined  MaxCount=255  InitialCount=0  Output=Count and Hit  HitValue=32  ResetInput=on  SamplesPerFrame=1  Ts=1  CntDtype=double  HitDtype=Logical
  D Flip-Flop : simulink_extras/Flip Flops/D Flip-Flop
  D Flip-Flop1 : simulink_extras/Flip Flops/D Flip-Flop
  Data Type Conversion1 : DataTypeConversion  OutDataTypeStr=boolean
  Data Type Conversion2 : DataTypeConversion  OutDataTypeStr=boolean
  Gain1 : Gain  Gain=-2
  Gain2 : Gain  Gain=2
  Play /Pausa : Subsystem
  Play/Pausa : Subsystem
  Pulse Generator1 : DiscretePulseGenerator  PulseType=Time based  Period=0.1  PulseWidth=50
  Pulse Generator3 : DiscretePulseGenerator  PulseType=Time based  Period=0.1  PulseWidth=50
  Saturation : Saturate  UpperLimit=180  LowerLimit=0
  Sum1 : Sum  Inputs=+|+
  Switch : Switch  Criteria=u2 > Threshold  Threshold=0.5  OutDataTypeStr=single  InputSameDT=on
  Switch6 : Switch  Criteria=u2 > Threshold  Threshold=0.5  OutDataTypeStr=single  InputSameDT=on
  Out : Outport
  wires:
  Counter1/1 -> Gain2/1
  Constant/1 -> Switch/1
  Constant9/1 -> Switch/3
  Constant2/1 -> Switch6/1
  Counter2/1 -> Gain1/1
  Gain1/1 -> Sum1/2
  D Flip-Flop1/1 -> Counter2/1
  Switch6/1 -> Data Type Conversion2/1
  Data Type Conversion2/1 -> D Flip-Flop1/1
  Pulse Generator3/1 -> D Flip-Flop1/3
  Constant19/1 -> Switch6/3
  In/1 -> Switch/2
  Saturation/1 -> Out/1
  Pulse Generator1/1 -> D Flip-Flop/3
  Sum1/1 -> Saturation/1
  Gain2/1 -> Sum1/1
  D Flip-Flop/1 -> Counter1/1
  Data Type Conversion1/1 -> D Flip-Flop/1
  Switch/1 -> Data Type Conversion1/1
  In1/1 -> Switch6/2
  Play/Pausa/1(CLK) -> D Flip-Flop/2
  Play /Pausa/1(CLK) -> D Flip-Flop1/2
  A/1 -> Play /Pausa/1(A), Play/Pausa/1(A)
  Y/1 -> Play /Pausa/2(Y), Play/Pausa/2(Y)
  B/1 -> Counter1/2, Counter2/2

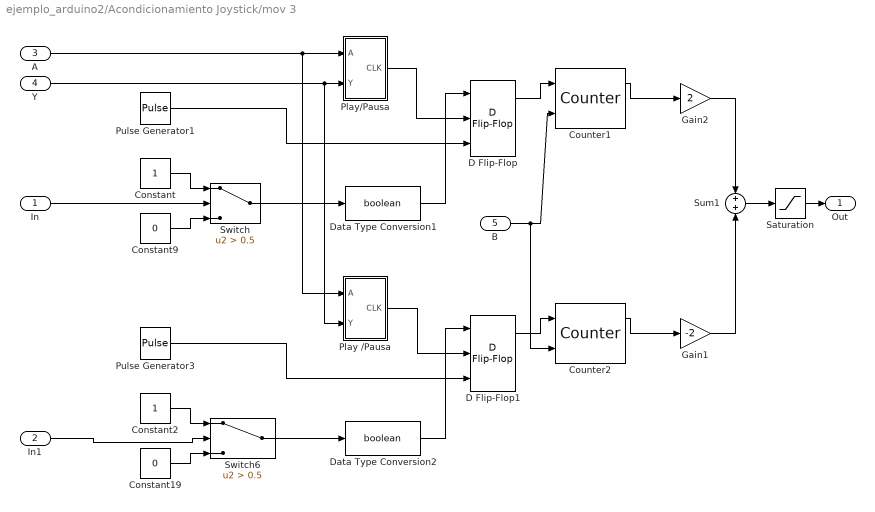
== system ejemplo_arduino2/Acondicionamiento Joystick/mov 3 ==
  In : Inport
  In1 : Inport  Port=2
  A : Inport  Port=3
  Y : Inport  Port=4
  B : Inport  Port=5
  Constant : Constant
  Constant19 : Constant  Value=0
  Constant2 : Constant
  Constant9 : Constant  Value=0
  Counter1 : dspswit3/Counter  Direction=Up  CountEvent=Rising edge  CounterSize=User defined  MaxCount=255  InitialCount=0  Output=Count and Hit  HitValue=32  ResetInput=on  SamplesPerFrame=1  Ts=1  CntDtype=double  HitDtype=Logical
  Counter2 : dspswit3/Counter  Direction=Up  CountEvent=Rising edge  CounterSize=User defined  MaxCount=255  InitialCount=0  Output=Count and Hit  HitValue=32  ResetInput=on  SamplesPerFrame=1  Ts=1  CntDtype=double  HitDtype=Logical
  D Flip-Flop : simulink_extras/Flip Flops/D Flip-Flop
  D Flip-Flop1 : simulink_extras/Flip Flops/D Flip-Flop
  Data Type Conversion1 : DataTypeConversion  OutDataTypeStr=boolean
  Data Type Conversion2 : DataTypeConversion  OutDataTypeStr=boolean
  Gain1 : Gain  Gain=-2
  Gain2 : Gain  Gain=2
  Play /Pausa : Subsystem
  Play/Pausa : Subsystem
  Pulse Generator1 : DiscretePulseGenerator  PulseType=Time based  Period=0.1  PulseWidth=50
  Pulse Generator3 : DiscretePulseGenerator  PulseType=Time based  Period=0.1  PulseWidth=50
  Saturation : Saturate  UpperLimit=180  LowerLimit=0
  Sum1 : Sum  Inputs=+|+
  Switch : Switch  Criteria=u2 > Threshold  Threshold=0.5  OutDataTypeStr=single  InputSameDT=on
  Switch6 : Switch  Criteria=u2 > Threshold  Threshold=0.5  OutDataTypeStr=single  InputSameDT=on
  Out : Outport
  wires:
  Counter1/1 -> Gain2/1
  Constant/1 -> Switch/1
  Constant9/1 -> Switch/3
  Constant2/1 -> Switch6/1
  Counter2/1 -> Gain1/1
  Gain1/1 -> Sum1/2
  D Flip-Flop1/1 -> Counter2/1
  Switch6/1 -> Data Type Conversion2/1
  Data Type Conversion2/1 -> D Flip-Flop1/1
  Pulse Generator3/1 -> D Flip-Flop1/3
  Constant19/1 -> Switch6/3
  In/1 -> Switch/2
  Saturation/1 -> Out/1
  Pulse Generator1/1 -> D Flip-Flop/3
  Sum1/1 -> Saturation/1
  Gain2/1 -> Sum1/1
  D Flip-Flop/1 -> Counter1/1
  Data Type Conversion1/1 -> D Flip-Flop/1
  Switch/1 -> Data Type Conversion1/1
  In1/1 -> Switch6/2
  Play/Pausa/1(CLK) -> D Flip-Flop/2
  Play /Pausa/1(CLK) -> D Flip-Flop1/2
  A/1 -> Play /Pausa/1(A), Play/Pausa/1(A)
  Y/1 -> Play /Pausa/2(Y), Play/Pausa/2(Y)
  B/1 -> Counter1/2, Counter2/2

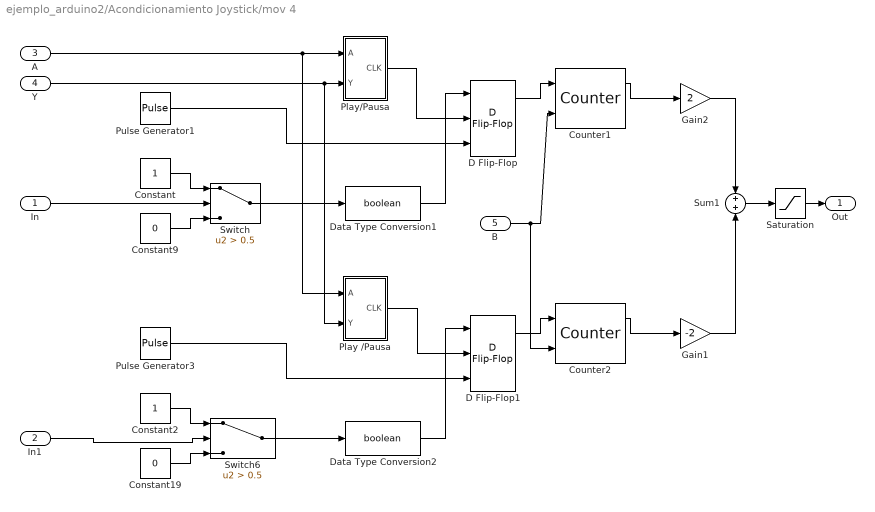
== system ejemplo_arduino2/Acondicionamiento Joystick/mov 4 ==
  In : Inport
  In1 : Inport  Port=2
  A : Inport  Port=3
  Y : Inport  Port=4
  B : Inport  Port=5
  Constant : Constant
  Constant19 : Constant  Value=0
  Constant2 : Constant
  Constant9 : Constant  Value=0
  Counter1 : dspswit3/Counter  Direction=Up  CountEvent=Rising edge  CounterSize=User defined  MaxCount=255  InitialCount=0  Output=Count and Hit  HitValue=32  ResetInput=on  SamplesPerFrame=1  Ts=1  CntDtype=double  HitDtype=Logical
  Counter2 : dspswit3/Counter  Direction=Up  CountEvent=Rising edge  CounterSize=User defined  MaxCount=255  InitialCount=0  Output=Count and Hit  HitValue=32  ResetInput=on  SamplesPerFrame=1  Ts=1  CntDtype=double  HitDtype=Logical
  D Flip-Flop : simulink_extras/Flip Flops/D Flip-Flop
  D Flip-Flop1 : simulink_extras/Flip Flops/D Flip-Flop
  Data Type Conversion1 : DataTypeConversion  OutDataTypeStr=boolean
  Data Type Conversion2 : DataTypeConversion  OutDataTypeStr=boolean
  Gain1 : Gain  Gain=-2
  Gain2 : Gain  Gain=2
  Play /Pausa : Subsystem
  Play/Pausa : Subsystem
  Pulse Generator1 : DiscretePulseGenerator  PulseType=Time based  Period=0.1  PulseWidth=50
  Pulse Generator3 : DiscretePulseGenerator  PulseType=Time based  Period=0.1  PulseWidth=50
  Saturation : Saturate  UpperLimit=180  LowerLimit=0
  Sum1 : Sum  Inputs=+|+
  Switch : Switch  Criteria=u2 > Threshold  Threshold=0.5  OutDataTypeStr=single  InputSameDT=on
  Switch6 : Switch  Criteria=u2 > Threshold  Threshold=0.5  OutDataTypeStr=single  InputSameDT=on
  Out : Outport
  wires:
  Counter1/1 -> Gain2/1
  Constant/1 -> Switch/1
  Constant9/1 -> Switch/3
  Constant2/1 -> Switch6/1
  Counter2/1 -> Gain1/1
  Gain1/1 -> Sum1/2
  D Flip-Flop1/1 -> Counter2/1
  Switch6/1 -> Data Type Conversion2/1
  Data Type Conversion2/1 -> D Flip-Flop1/1
  Pulse Generator3/1 -> D Flip-Flop1/3
  Constant19/1 -> Switch6/3
  In/1 -> Switch/2
  Saturation/1 -> Out/1
  Pulse Generator1/1 -> D Flip-Flop/3
  Sum1/1 -> Saturation/1
  Gain2/1 -> Sum1/1
  D Flip-Flop/1 -> Counter1/1
  Data Type Conversion1/1 -> D Flip-Flop/1
  Switch/1 -> Data Type Conversion1/1
  In1/1 -> Switch6/2
  Play/Pausa/1(CLK) -> D Flip-Flop/2
  Play /Pausa/1(CLK) -> D Flip-Flop1/2
  A/1 -> Play /Pausa/1(A), Play/Pausa/1(A)
  Y/1 -> Play /Pausa/2(Y), Play/Pausa/2(Y)
  B/1 -> Counter1/2, Counter2/2

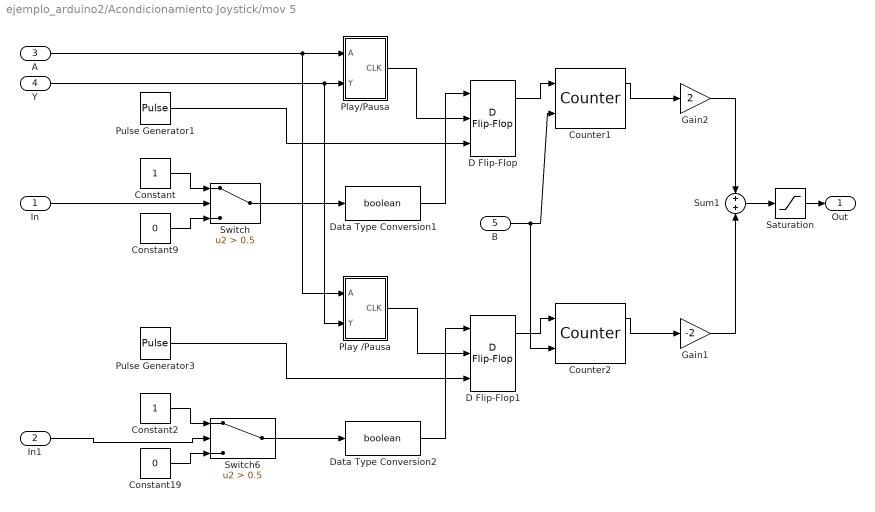
== system ejemplo_arduino2/Acondicionamiento Joystick/mov 5 ==
  In : Inport
  In1 : Inport  Port=2
  A : Inport  Port=3
  Y : Inport  Port=4
  B : Inport  Port=5
  Constant : Constant
  Constant19 : Constant  Value=0
  Constant2 : Constant
  Constant9 : Constant  Value=0
  Counter1 : dspswit3/Counter  Direction=Up  CountEvent=Rising edge  CounterSize=User defined  MaxCount=255  InitialCount=0  Output=Count and Hit  HitValue=32  ResetInput=on  SamplesPerFrame=1  Ts=1  CntDtype=double  HitDtype=Logical
  Counter2 : dspswit3/Counter  Direction=Up  CountEvent=Rising edge  CounterSize=User defined  MaxCount=255  InitialCount=0  Output=Count and Hit  HitValue=32  ResetInput=on  SamplesPerFrame=1  Ts=1  CntDtype=double  HitDtype=Logical
  D Flip-Flop : simulink_extras/Flip Flops/D Flip-Flop
  D Flip-Flop1 : simulink_extras/Flip Flops/D Flip-Flop
  Data Type Conversion1 : DataTypeConversion  OutDataTypeStr=boolean
  Data Type Conversion2 : DataTypeConversion  OutDataTypeStr=boolean
  Gain1 : Gain  Gain=-2
  Gain2 : Gain  Gain=2
  Play /Pausa : Subsystem
  Play/Pausa : Subsystem
  Pulse Generator1 : DiscretePulseGenerator  PulseType=Time based  Period=0.1  PulseWidth=50
  Pulse Generator3 : DiscretePulseGenerator  PulseType=Time based  Period=0.1  PulseWidth=50
  Saturation : Saturate  UpperLimit=180  LowerLimit=0
  Sum1 : Sum  Inputs=+|+
  Switch : Switch  Criteria=u2 > Threshold  Threshold=0.5  OutDataTypeStr=single  InputSameDT=on
  Switch6 : Switch  Criteria=u2 > Threshold  Threshold=0.5  OutDataTypeStr=single  InputSameDT=on
  Out : Outport
  wires:
  Counter1/1 -> Gain2/1
  Constant/1 -> Switch/1
  Constant9/1 -> Switch/3
  Constant2/1 -> Switch6/1
  Counter2/1 -> Gain1/1
  Gain1/1 -> Sum1/2
  D Flip-Flop1/1 -> Counter2/1
  Switch6/1 -> Data Type Conversion2/1
  Data Type Conversion2/1 -> D Flip-Flop1/1
  Pulse Generator3/1 -> D Flip-Flop1/3
  Constant19/1 -> Switch6/3
  In/1 -> Switch/2
  Saturation/1 -> Out/1
  Pulse Generator1/1 -> D Flip-Flop/3
  Sum1/1 -> Saturation/1
  Gain2/1 -> Sum1/1
  D Flip-Flop/1 -> Counter1/1
  Data Type Conversion1/1 -> D Flip-Flop/1
  Switch/1 -> Data Type Conversion1/1
  In1/1 -> Switch6/2
  Play/Pausa/1(CLK) -> D Flip-Flop/2
  Play /Pausa/1(CLK) -> D Flip-Flop1/2
  A/1 -> Play /Pausa/1(A), Play/Pausa/1(A)
  Y/1 -> Play /Pausa/2(Y), Play/Pausa/2(Y)
  B/1 -> Counter1/2, Counter2/2
